simulink model "Radar_Signal_Processing"  (R2021b)
settings: Solver=VariableStepAuto  StartTime=0.0  StopTime=stop_time  RelTol=1e-3
values from neighbouring files (symbols this model uses):
  num_samples_in_sampling_period = obj.ADC_Samples    [Radar.m]
  num_samples_prior_to_sample_period = int32((obj.ADC_ValidStartTime_us + obj.IdleTime_us) *                 obj.ADC_SampleRate_MSps)    [Radar.m]
  simulator = Simulator_revB()    [compute_sensed_targets.m]    (also in compute_sensed_values.m)
undefined symbols (not defined in the file or in its folder): designMultirateFIR, magnitude, physconst
libraries: phaseddetectlib x5, simulink x1, radarlib x1, dspmlti4 x1
settings Model: Creator=David  LastModifiedBy=David

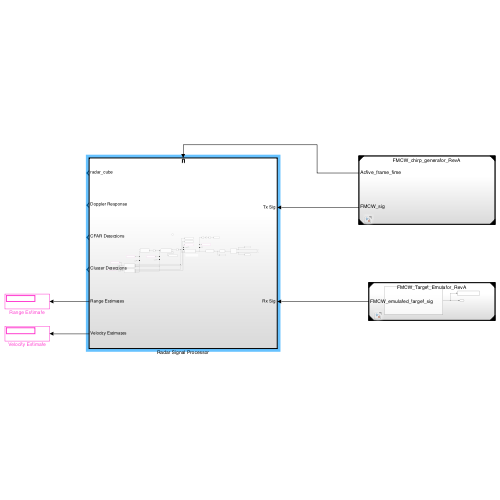
[thumbnail: Simulink's stored preview of the top-level diagram]
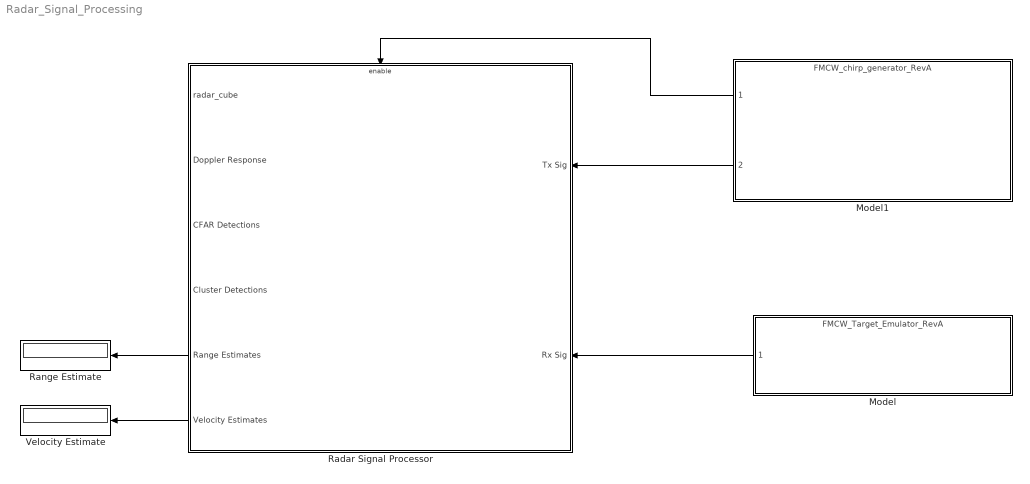
== system Radar_Signal_Processing ==
  Model : ModelReference  ModelNameDialog=FMCW_Target_Emulator_RevA.slx  ModelReferenceVersion=1.18
  Model1 : ModelReference  ModelNameDialog=FMCW_chirp_generator_RevA.slx  ModelReferenceVersion=1.12
  Radar Signal Processor : Subsystem
  Range Estimate : Display
  Velocity Estimate : Display
  wires:
  Model1/2 -> Radar Signal Processor/1(Tx Sig)
  Model/1 -> Radar Signal Processor/2(Rx Sig)
  Radar Signal Processor/6(Velocity Estimates) -> Velocity Estimate/1
  Radar Signal Processor/5(Range Estimates) -> Range Estimate/1
  Model1/1 -> Radar Signal Processor/Enable

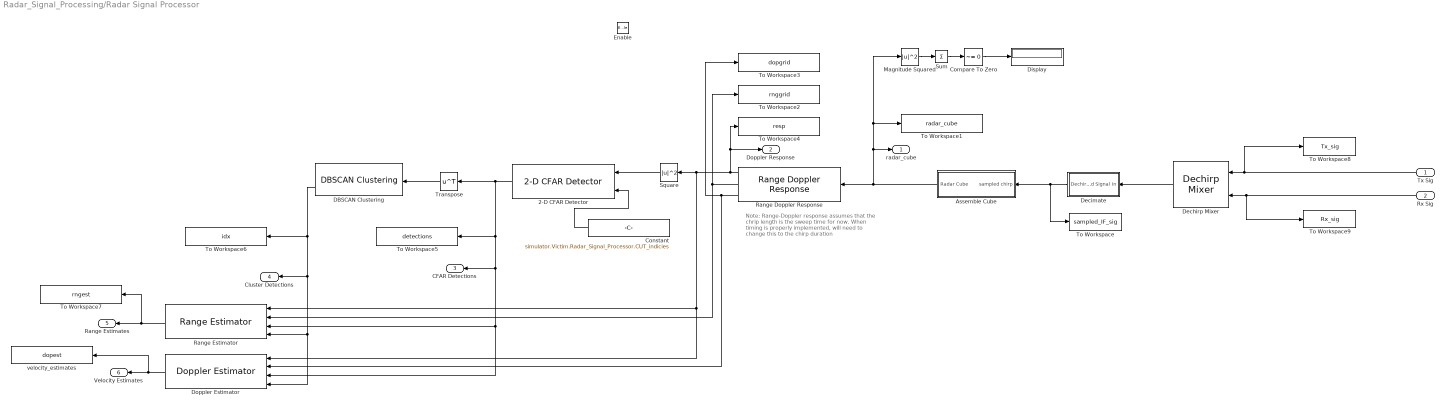
== system Radar_Signal_Processing/Radar Signal Processor ==
  note: Note: Range-Doppler response assumes
      | that the chrip length is the sweep time
      | for now. When timing is properly implemented,
      | will need to change this to the chirp duration
  Tx Sig : Inport
  Rx Sig : Inport  Port=2
  Enable : EnablePort
  2-D CFAR Detector : phaseddetectlib/2-D CFAR Detector  Method=CA  Rank=1  GuardBandSize=simulator.Victim.Radar_Signal_Processor.guard_region  TrainingBandSize=simulator.Victim.Radar_Signal_Processor.training_region  ThresholdFactor=Auto  ProbabilityFalseAlarm=simulator.Victim.Radar_Signal_Processor.PFAR  CustomThresholdFactor=1  OutputFormat=Detection index  ThresholdOutputPort=off  NoisePowerOutputPort=off  NumDetectionsSource=Auto  NumDetections=1  SimulateUsing=Interpreted execution
      settings: SourceProductBaseCode=AR
  Assemble Cube : Subsystem
  Compare To Zero : simulink/Logic and Bit Operations/Compare To Zero  relop=~=  OutDataTypeStr=boolean
  Constant : Constant  Value=simulator.Victim.Radar_Signal_Processor.CUT_indicies  VectorParams1D=off
  DBSCAN Clustering : radarlib/DBSCAN Clustering  BlockOutputs=Index and Cluster ID  EpsilonSource=Property  Epsilon=simulator.Victim.Radar_Signal_Processor.Epsilon  MinNumPoints=simulator.Victim.Radar_Signal_Processor.minpts  MaxNumPoints=10  EpsilonHistoryLength=10  EnableDisambiguation=off  AmbiguousDimension=1  SimulateUsing=Interpreted execution
      settings: SourceProductBaseCode=RA
  Dechirp Mixer : phaseddetectlib/Dechirp Mixer
      settings: SourceProductBaseCode=AR
  Decimate : Subsystem
  Display : Display
  Doppler Estimator : phaseddetectlib/Doppler Estimator  NumEstimatesSource=Property  NumEstimates=simulator.Victim.Radar_Signal_Processor.NumEstimates_dplr  VarianceOutputPort=off  NumPulses=2  NoisePowerSource=Property  NoisePower=1  ClusterInputPort=on  SimulateUsing=Interpreted execution
      settings: SourceProductBaseCode=AR
  Magnitude Squared : Math  Operator=magnitude^2  SaturateOnIntegerOverflow=on
  Range Doppler Response : phaseddetectlib/Range Doppler Response  RangeMethod=FFT  PropagationSpeed=physconst( 'lightspeed' )  SampleRateFromInputCheckbox=off  SampleRate=simulator.Victim.ADC_SampleRate_MSps * 1e6  SweepSlope=simulator.Victim.FrequencySlope_MHz_us * 1e12  DechirpInput=off  RangeFFTLengthSource=Auto  RangeFFTLength=1024  RangeWindow=Hann  RangeSidelobeAttenuation=30  CustomRangeWindow=@hamming  ReferenceRangeCentered=off  ReferenceRange=0  MaximumNumInputSamplesSource=Auto  MaximumNumInputSamples=100  PRFSource=Property  PRF=1 / (simulator.Victim.ChirpCycleTime_us *1e-6)  DopplerFFTLengthSource=Property  DopplerFFTLength=simulator.Victim.NumChirps  DopplerWindow=Hann  DopplerSidelobeAttenuation=30  CustomDopplerWindow=@hamming  DopplerOutput=Speed  OperatingFrequency=simulator.Victim.StartFrequency_GHz * 1e9  SimulateUsing=Code generation
      settings: SourceProductBaseCode=AR
  Range Estimator : phaseddetectlib/Range Estimator  NumEstimatesSource=Property  NumEstimates=simulator.Victim.Radar_Signal_Processor.NumEstimates_rng  VarianceOutputPort=off  RMSResolution=1  NoisePowerSource=Property  NoisePower=1  ClusterInputPort=on  SimulateUsing=Interpreted execution
      settings: SourceProductBaseCode=AR
  Square : Math  Operator=magnitude^2  SaturateOnIntegerOverflow=on
  Sum : Sum  Inputs=+
  To Workspace : ToWorkspace  VariableName=sampled_IF_sig  SampleTime=-1
      settings: MaxDataPoints=2
  To Workspace1 : ToWorkspace  VariableName=radar_cube  SampleTime=-1
      settings: MaxDataPoints=2
  To Workspace2 : ToWorkspace  VariableName=rnggrid  SampleTime=-1
      settings: MaxDataPoints=1
  To Workspace3 : ToWorkspace  VariableName=dopgrid  SampleTime=-1
      settings: MaxDataPoints=1
  To Workspace4 : ToWorkspace  VariableName=resp  SampleTime=-1
      settings: MaxDataPoints=2
  To Workspace5 : ToWorkspace  VariableName=detections  SampleTime=-1
      settings: MaxDataPoints=2
  To Workspace6 : ToWorkspace  VariableName=idx  SampleTime=-1
      settings: MaxDataPoints=2
  To Workspace7 : ToWorkspace  VariableName=rngest  SampleTime=-1
      settings: MaxDataPoints=2
  To Workspace8 : ToWorkspace  VariableName=Tx_sig  SampleTime=-1
      settings: MaxDataPoints=2
  To Workspace9 : ToWorkspace  VariableName=Rx_sig  SampleTime=-1
      settings: MaxDataPoints=2
  Transpose : Math  Operator=transpose  SaturateOnIntegerOverflow=on
  velocity_estimates : ToWorkspace  VariableName=dopest  SampleTime=-1
      settings: MaxDataPoints=2
  radar_cube : Outport
  Doppler Response : Outport  Port=2
  CFAR Detections : Outport  Port=3
  Cluster Detections : Outport  Port=4
  Range Estimates : Outport  Port=5
  Velocity Estimates : Outport  Port=6
  wires:
  Compare To Zero/1 -> Display/1
  Magnitude Squared/1 -> Sum/1
  Sum/1 -> Compare To Zero/1
  Tx Sig/1 -> To Workspace8/1, Dechirp Mixer/1
  Rx Sig/1 -> To Workspace9/1, Dechirp Mixer/2
  Decimate/1(Dechirped Signal) -> Assemble Cube/1(sampled chirp), To Workspace/1
  Dechirp Mixer/1 -> Decimate/1(In)
  DBSCAN Clustering/2 -> To Workspace6/1, Cluster Detections/1, Doppler Estimator/4, Range Estimator/4
  Assemble Cube/1(Radar Cube) -> Magnitude Squared/1, To Workspace1/1, radar_cube/1, Range Doppler Response/1
  2-D CFAR Detector/1 -> Transpose/1, To Workspace5/1, CFAR Detections/1, Doppler Estimator/3, Range Estimator/3
  Range Doppler Response/1 -> To Workspace4/1, Doppler Response/1, Doppler Estimator/1, Range Estimator/1, Square/1
  Square/1 -> 2-D CFAR Detector/1
  Transpose/1 -> DBSCAN Clustering/1
  Range Estimator/1 -> To Workspace7/1, Range Estimates/1
  Constant/1 -> 2-D CFAR Detector/2
  Doppler Estimator/1 -> velocity_estimates/1, Velocity Estimates/1
  Range Doppler Response/2 -> Range Estimator/2, To Workspace2/1
  Range Doppler Response/3 -> Doppler Estimator/2, To Workspace3/1

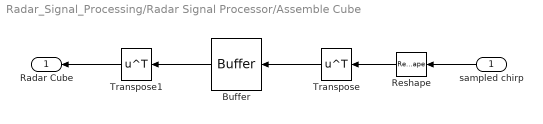
== system Radar_Signal_Processing/Radar Signal Processor/Assemble Cube ==
  sampled chirp : Inport
  Buffer : Buffer  N=simulator.Victim.NumChirps  OutputFrames=off
  Reshape : Reshape
  Transpose : Math  Operator=transpose  SaturateOnIntegerOverflow=on
  Transpose1 : Math  Operator=transpose  SaturateOnIntegerOverflow=on
  Radar Cube : Outport
  wires:
  sampled chirp/1 -> Reshape/1
  Transpose/1 -> Buffer/1
  Buffer/1 -> Transpose1/1
  Transpose1/1 -> Radar Cube/1
  Reshape/1 -> Transpose/1

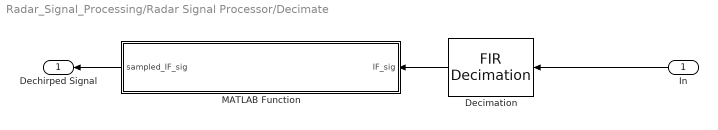
== system Radar_Signal_Processing/Radar Signal Processor/Decimate ==
  In : Inport
  Decimation : dspmlti4/FIR Decimation  FilterSource=Auto  h=designMultirateFIR(1,2)  D=simulator.Victim.Radar_Signal_Processor.decimation_factor  filtStruct=Direct form  FilterObject=simulator.Victim.low_pass_filter  InputProcessing=Columns as channels (frame based)  framing=Enforce single-rate processing  inputOffset=0  outputBufInitCond=0  roundingMode=Floor  overflowMode=off  firstCoeffDataTypeStr=Inherit: Same word length as input  firstCoeffMin=[]  firstCoeffMax=[]  firstCoeffLastDataTypeStr=Inherit: Same word length as input  outputDataTypeStr=Inherit: Same as accumulator  outputMin=[]  outputMax=[]  outputLastDataTypeStr=Inherit: Same as accumulator
  MATLAB Function : MATLAB Function  TreatAsAtomicUnit=on
  Dechirped Signal : Outport
  wires:
  Decimation/1 -> MATLAB Function/1(IF_sig)
  MATLAB Function/1(sampled_IF_sig) -> Dechirped Signal/1
  In/1 -> Decimation/1

== matlab function Radar_Signal_Processing/Radar Signal Processor/Decimate/MATLAB Function ==
  data: IF_sig input; sampled_IF_sig output; num_samples_prior_to_sample_period parameter; num_samples_in_sampling_period parameter
function sampled_IF_sig = select_sampled_IF_sig(IF_sig,num_samples_prior_to_sample_period,num_samples_in_sampling_period)

    sampled_IF_sig = IF_sig(...
        num_samples_prior_to_sample_period + 1:...
        num_samples_prior_to_sample_period + num_samples_in_sampling_period);
